simulink model "HW2SPWM"  (R2024b)
settings: Solver=VariableStepAuto  StartTime=0.0  StopTime=2.0  MaxStep=10e-6  RelTol=1e-3
libraries: spsMeanLib x10, spsCurrentMeasurementLib x7, spsVoltageMeasurementLib x7, spsMosfetLib x6, simulink x3, spsTHDLib x2, spsDCVoltageSourceLib x1, spsGroundLib x1, spsThreePhaseSeriesRLCBranchLib x1, spsThreePhaseVIMeasurementLib x1, spsTriangleGeneratorLib x1, spspowerguiLib x1
settings Model: Creator=joekr  LastModifiedBy=joekr
settings DataIOCC: SaveOutput=off  SignalLogging=off  DSMLogging=off  SaveTime=off  ReturnWorkspaceOutputs=off

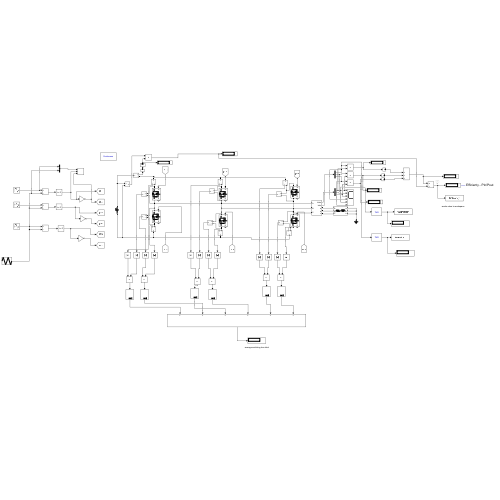
[thumbnail: Simulink's stored preview of the top-level diagram]
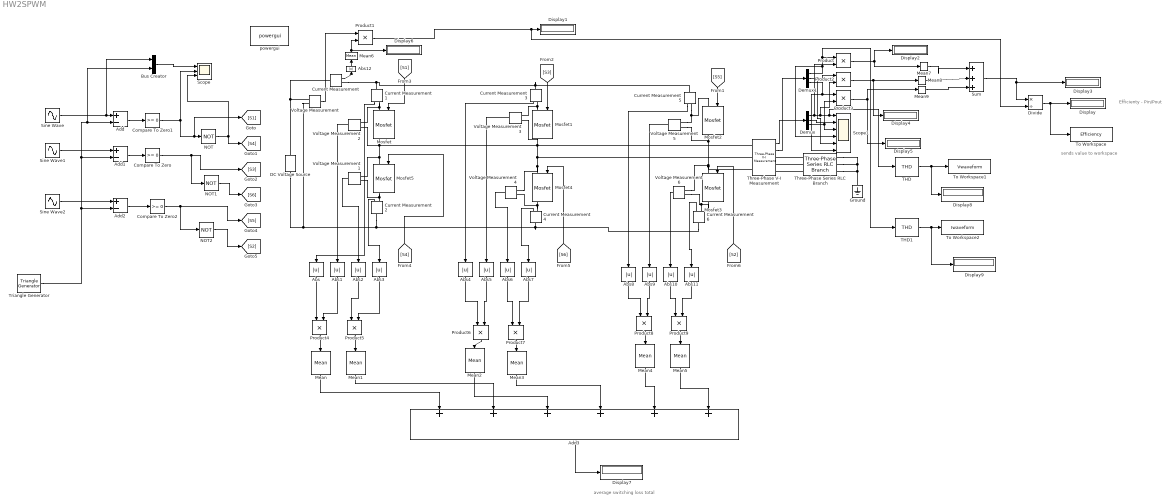
== system HW2SPWM ==
  note: sends value to workspace
  note: average switching loss total
  note: Efficienty - Pin/Pout
  Abs{,1..12} (13 alike) : Abs  SaturateOnIntegerOverflow=off
  Add : Sum  Inputs=+-
  Add1 : Sum  Inputs=+-
  Add2 : Sum  Inputs=+-
  Add3 : Sum  Inputs=++++++
  Bus Creator : BusCreator  Inputs=2
  Compare To Zero : simulink/Logic and Bit Operations/Compare To Zero  relop=>=  OutDataTypeStr=boolean
  Compare To Zero1 : simulink/Logic and Bit Operations/Compare To Zero  relop=>=  OutDataTypeStr=boolean
  Compare To Zero2 : simulink/Logic and Bit Operations/Compare To Zero  relop=>=  OutDataTypeStr=boolean
  Current Measurement{,1..6} (7 alike) : spsCurrentMeasurementLib/Current Measurement  PhasorSimulation=off  OutputType=Complex  PSBequivalent=0
  DC Voltage Source : spsDCVoltageSourceLib/DC Voltage Source  Amplitude=200  Measurements=None
  Demux : Demux  Outputs=3
  Demux1 : Demux  Outputs=3
  Display{,1..9} (10 alike) : Display
  Divide : Product  Inputs=*/
  Ground : spsGroundLib/Ground  LConnTagsString=a
  Mean{,1..9} (10 alike) : spsMeanLib/Mean  Freq=60  Vinit=0  Ts=0
  Mosfet{,1..5} (6 alike) : spsMosfetLib/Mosfet  Ron=0.1  Lon=0  Rd=0.01  Vfd=0  IC=0  Rs=1e5  Cs=inf  Measurements=on
  NOT : Logic  Operator=NOT  IconShape=distinctive  AllPortsSameDT=off  OutDataTypeStr=boolean
  NOT1 : Logic  Operator=NOT  IconShape=distinctive  AllPortsSameDT=off  OutDataTypeStr=boolean
  NOT2 : Logic  Operator=NOT  IconShape=distinctive  AllPortsSameDT=off  OutDataTypeStr=boolean
  Product{,1..9} (10 alike) : Product
  Scope : Scope  NumInputPorts=3
  Scope1 : Scope  NumInputPorts=6
  Sine Wave : Sin  Amplitude=0.9  Frequency=120*pi  SampleTime=0
  Sine Wave1 : Sin  Amplitude=0.9  Frequency=120*pi  Phase=2*pi/3  SampleTime=0
  Sine Wave2 : Sin  Amplitude=0.9  Frequency=120*pi  Phase=4*pi/3  SampleTime=0
  Sum : Sum  Inputs=|+++
  THD : spsTHDLib/THD  Freq=60  Ts=0
  THD1 : spsTHDLib/THD  Freq=60  Ts=0
  Three-Phase Series RLC Branch : spsThreePhaseSeriesRLCBranchLib/Three-Phase Series RLC Branch  LConnTagsString=A|B|C  RConnTagsString=A|B|C  BranchType=RL  Resistance=10  Inductance=0.1  Capacitance=1e-6  Measurements=None
  Three-Phase V-I Measurement : spsThreePhaseVIMeasurementLib/Three-Phase V-I Measurement  VoltageMeasurement=phase-to-ground  SetLabelV=off  LabelV=Vabc  Vpu=off  VpuLL=off  CurrentMeasurement=yes  SetLabelI=off  LabelI=Iabc  Ipu=off  Pbase=100e6  Vbase=500e3  OutputType=Complex  PhasorSimulation=off  PSBequivalent=0
  To Workspace : ToWorkspace  VariableName=Efficiency  SaveFormat=Structure With Time  SampleTime=-1
  To Workspace1 : ToWorkspace  VariableName=Vwaveform  SaveFormat=Structure With Time  SampleTime=-1
  To Workspace2 : ToWorkspace  VariableName=Iwaveform  SaveFormat=Structure With Time  SampleTime=-1
  Triangle Generator : spsTriangleGeneratorLib/Triangle Generator  Freq=600  Phase=90  Ts=0
  Voltage Measurement{,1..6} (7 alike) : spsVoltageMeasurementLib/Voltage Measurement  PhasorSimulation=off  OutputType=Complex  PSBequivalent=0
  powergui : spspowerguiLib/powergui  Priority=1  SimulationMode=Continuous  SampleTime=50e-6  frequency=60  Iterations=50  frequencyindice=0  Pbase=100e6  ErrMax=1e-4  UnitsV=kV  UnitsW=MW  buscounter=0  FunctionMessages=off  echomessages=off  EnableUseOfTLC=off  CurrentSourceSwitches=off  DisableSnubberDevices=off  DisableRonSwitches=off  DisableVfSwitches=off  DisplayEquations=off  AutomaticDiscreteSolvers=off  SolverType=Tustin/Backward Euler (TBE)  Interpol=off  ExternalGateDelay=off  methode=off  Ts=100  x0status=blocks  SPID=on  SwTol=0  HookPort=off  NonlinearTolerance=1e-4  nMaxIteration=100  ContinueOnMaxIteration=off  RestoreLinks=warning  ResistiveCurrentMeasurement=off  Frange=[0:2:500]  Ylog=off  Xlog=on  ShowGrid=off  save=off  variable=ZData  structure=0  ZoomFFT=off  StartTime=0.0  cycles=1  DisplayStyle=1  fundamental=60  FreqAxis=off  MaxFrequency=1000  frequencyindicesteady=1  RmsSteady=1  display=off
  wires:
  Triangle Generator/1 -> Bus Creator/2, Add/2, Add1/2, Add2/2
  Sine Wave2/1 -> Add2/1
  Sine Wave1/1 -> Add1/1
  Sine Wave/1 -> Bus Creator/1, Add/1
  Bus Creator/1 -> Scope/1
  NOT/1 -> Scope/3, [S4]
  NOT2/1 -> [S2]
  NOT1/1 -> [S6]
  Add1/1 -> Compare To Zero/1
  Compare To Zero/1 -> NOT1/1, [S3]
  Add/1 -> Compare To Zero1/1
  Compare To Zero1/1 -> Scope/2, [S1], NOT/1
  Compare To Zero2/1 -> NOT2/1, [S5]
  Add2/1 -> Compare To Zero2/1
  [S1] -> Mosfet/1
  [S4] -> Mosfet5/1
  [S6] -> Mosfet4/1
  [S2] -> Mosfet3/1
  [S3] -> Mosfet1/1
  [S5] -> Mosfet2/1
  Three-Phase V-I Measurement/1 -> Demux/1
  Demux/1 -> Product/2, Product2/2, THD/1, Scope1/1
  Demux/2 -> Scope1/2
  Demux/3 -> Product3/2, Scope1/3
  Three-Phase V-I Measurement/2 -> Demux1/1
  Demux1/1 -> THD1/1, Product/1, Scope1/4
  Voltage Measurement/1 -> Product1/1
  Divide/1 -> To Workspace/1, Display/1
  Demux1/2 -> Product2/1, Scope1/5
  Demux1/3 -> Product3/1, Scope1/6
  Product/1 -> Mean7/1, Display2/1
  Product2/1 -> Mean8/1, Display4/1
  Product3/1 -> Mean9/1, Display5/1
  Product6/1 -> Mean2/1
  Product7/1 -> Mean3/1
  Product5/1 -> Mean1/1
  Product4/1 -> Mean/1
  Mean/1 -> Add3/1
  Mean1/1 -> Add3/2
  Mean2/1 -> Add3/3
  Mean3/1 -> Add3/4
  Mean4/1 -> Add3/5
  Mean5/1 -> Add3/6
  Product8/1 -> Mean4/1
  Product9/1 -> Mean5/1
  Add3/1 -> Display7/1
  Current Measurement1/1 -> Abs/1
  Voltage Measurement2/1 -> Abs1/1
  Voltage Measurement1/1 -> Abs2/1
  Current Measurement2/1 -> Abs3/1
  Abs/1 -> Product4/1
  Abs1/1 -> Product4/2
  Abs2/1 -> Product5/1
  Abs3/1 -> Product5/2
  Current Measurement3/1 -> Abs4/1
  Voltage Measurement3/1 -> Abs5/1
  Voltage Measurement4/1 -> Abs6/1
  Current Measurement4/1 -> Abs7/1
  Current Measurement6/1 -> Abs11/1
  Voltage Measurement6/1 -> Abs10/1
  Voltage Measurement5/1 -> Abs9/1
  Current Measurement5/1 -> Abs8/1
  Abs4/1 -> Product6/1
  Abs5/1 -> Product6/2
  Abs6/1 -> Product7/1
  Abs7/1 -> Product7/2
  Abs8/1 -> Product8/1
  Abs9/1 -> Product8/2
  Abs10/1 -> Product9/1
  Abs11/1 -> Product9/2
  Sum/1 -> Divide/1, Display3/1
  Mean7/1 -> Sum/1
  Mean8/1 -> Sum/2
  Mean9/1 -> Sum/3
  Product1/1 -> Divide/2, Display1/1
  Mean6/1 -> Product1/2, Display6/1
  Current Measurement/1 -> Abs12/1
  Abs12/1 -> Mean6/1
  THD/1 -> Display8/1, To Workspace1/1
  THD1/1 -> Display9/1, To Workspace2/1
  connections:
  Current Measurement5/LConn1 -- Current Measurement3/LConn1 -- Current Measurement/RConn1 -- Current Measurement1/LConn1
  DC Voltage Source/LConn1 -- Current Measurement6/LConn1 -- Current Measurement4/LConn1 -- Current Measurement2/LConn1 -- Voltage Measurement/LConn2
  Mosfet/RConn1 -- Voltage Measurement1/LConn1 -- Mosfet5/LConn1 -- Voltage Measurement2/LConn2 -- Three-Phase V-I Measurement/LConn1
  Mosfet1/RConn1 -- Voltage Measurement3/LConn2 -- Three-Phase V-I Measurement/LConn2 -- Voltage Measurement4/LConn1 -- Mosfet4/LConn1
  Mosfet2/RConn1 -- Voltage Measurement6/LConn1 -- Three-Phase V-I Measurement/LConn3 -- Mosfet3/LConn1 -- Voltage Measurement5/LConn2
  Three-Phase Series RLC Branch/RConn3 -- Three-Phase Series RLC Branch/RConn1 -- Three-Phase Series RLC Branch/RConn2 -- Ground/LConn1
  Three-Phase Series RLC Branch/LConn1 -- Three-Phase V-I Measurement/RConn1
  Three-Phase Series RLC Branch/LConn2 -- Three-Phase V-I Measurement/RConn2
  Three-Phase Series RLC Branch/LConn3 -- Three-Phase V-I Measurement/RConn3
  DC Voltage Source/RConn1 -- Current Measurement/LConn1 -- Voltage Measurement/LConn1
  Mosfet/LConn1 -- Voltage Measurement2/LConn1 -- Current Measurement1/RConn1
  Current Measurement2/RConn1 -- Voltage Measurement1/LConn2 -- Mosfet5/RConn1
  Current Measurement3/RConn1 -- Voltage Measurement3/LConn1 -- Mosfet1/LConn1
  Mosfet4/RConn1 -- Voltage Measurement4/LConn2 -- Current Measurement4/RConn1
  Current Measurement5/RConn1 -- Voltage Measurement5/LConn1 -- Mosfet2/LConn1
  Mosfet3/RConn1 -- Voltage Measurement6/LConn2 -- Current Measurement6/RConn1
